simulink model "partial_acc_model_breach"  (R2017a)
settings: Solver=VariableStepAuto  StartTime=0.0  StopTime=tspan(end)  RelTol=1e-3
undefined symbols (not defined in the file): d0, ed0, ev0, nrad, v0, vl
settings Model: Creator=LuanNguyen  LastModifiedBy=LuanNguyen
settings DataIOCC: ExternalInput=[t__, u__]  LoadExternalInput=on  SaveFormat=StructureWithTime  ReturnWorkspaceOutputs=on

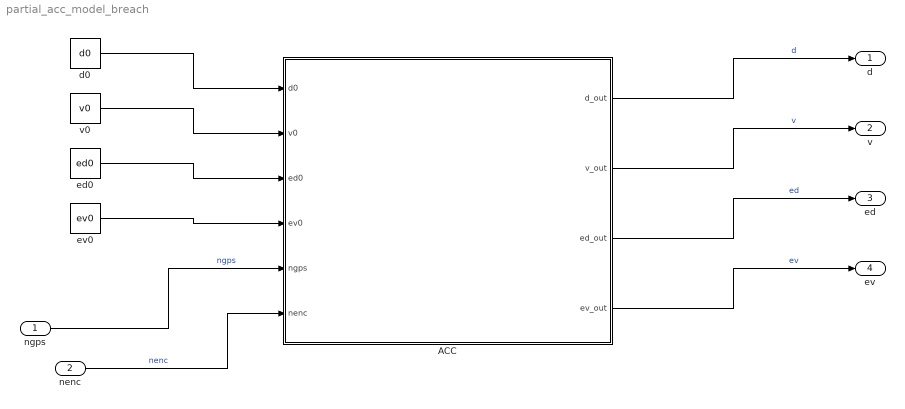
== system partial_acc_model_breach ==
  ngps : Inport
  nenc : Inport  Port=2
  ACC : Stateflow chart  TreatAsAtomicUnit=on
  d0 : Constant  Value=d0
  ed0 : Constant  Value=ed0
  ev0 : Constant  Value=ev0
  v0 : Constant  Value=v0
  d : Outport
  v : Outport  Port=2
  ed : Outport  Port=3
  ev : Outport  Port=4
  wires:
  ACC/1(d_out) -> d/1  "d"
  ACC/2(v_out) -> v/1  "v"
  ACC/3(ed_out) -> ed/1  "ed"
  ACC/4(ev_out) -> ev/1  "ev"
  d0/1 -> ACC/1(d0)
  v0/1 -> ACC/2(v0)
  ed0/1 -> ACC/3(ed0)
  ev0/1 -> ACC/4(ev0)
  ngps/1 -> ACC/5(ngps)  "ngps"
  nenc/1 -> ACC/6(nenc)  "nenc"

== stateflow chart partial_acc_model_breach/ACC ==
  settings: updateMethod=CONTINUOUS
  state Spacing_Control
    du:
    d_dot = -v+vl;
    v_dot = 0.25*d - 2*v - 0.25*ed + ev - 0.25*(10 + 2*(v-ev))+2*vl;
    ed_dot = -10*ed - ev + nrad;
    ev_dot = -2*ev+0.5*(ngps + nenc);
    d_out = d;
    v_out = v;
    ed_out = ed;
    ev_out = ev;
  state Speed_Control
    du:
    d_dot = -v+vl;
    v_dot = -2*v+ev+2*vl;
    ed_dot = -10*ed - ev + nrad;
    ev_dot = -2*ev+0.5*(ngps + nenc);
    d_out = d;
    v_out = v;
    ed_out = ed;
    ev_out = ev;
  (default) -> Speed_Control : {d = d0; v = v0; ed = ed0; ev = ev0;}
  Speed_Control -> Spacing_Control : [d - ed < 10 + 2*(v-ev)]
  Spacing_Control -> Speed_Control : [d - ed >= 10 + 2*(v-ev)]
  data: ed local; ev local; v local; d_out output; v_out output; ed_out output; ev_out output; vl local double; nrad local double; d0 input double; v0 input double; ed0 input double; ev0 input double; d local; ngps input double; nenc input double
  data ed settings: updateMethod=SF_CONTINUOUS_TIME_DATA
  data ev settings: updateMethod=SF_CONTINUOUS_TIME_DATA
  data v settings: updateMethod=SF_CONTINUOUS_TIME_DATA
  data d settings: updateMethod=SF_CONTINUOUS_TIME_DATA
